simulink model "KP_Nikolaev_v27"  (R2021a)
settings: Solver=VariableStepAuto  StartTime=0.0  StopTime=50  RelTol=0.05
undefined symbols (not defined in the file): Angle, D11, Delta, Magnitude
libraries: spsThreePhaseBreakerLib x25, spsThreePhaseSeriesRLCLoadLib x15, spsSeriesRLCBranchLib x15, slrealtimeutilitieslib x14, slrealtimeiplib x13, spsThreePhaseVIMeasurementLib x6, spsCurrentMeasurementLib x3, spsPLLLib x3, spsVoltageMeasurementLib x3, spsExcitationSystemLib x2, spsSteamTurbineandGovernorLib x2, spsSynchronousMachinepuStandardLib x2
settings Model: Creator=kirill  LastModifiedBy=Артур
settings SolverCC: AlgebraicLoopSolver=TrustRegion
settings DebuggingCC: UnconnectedInputMsg=none  UnconnectedOutputMsg=none  UnconnectedLineMsg=none  SFMachineParentedDataDiag=warning

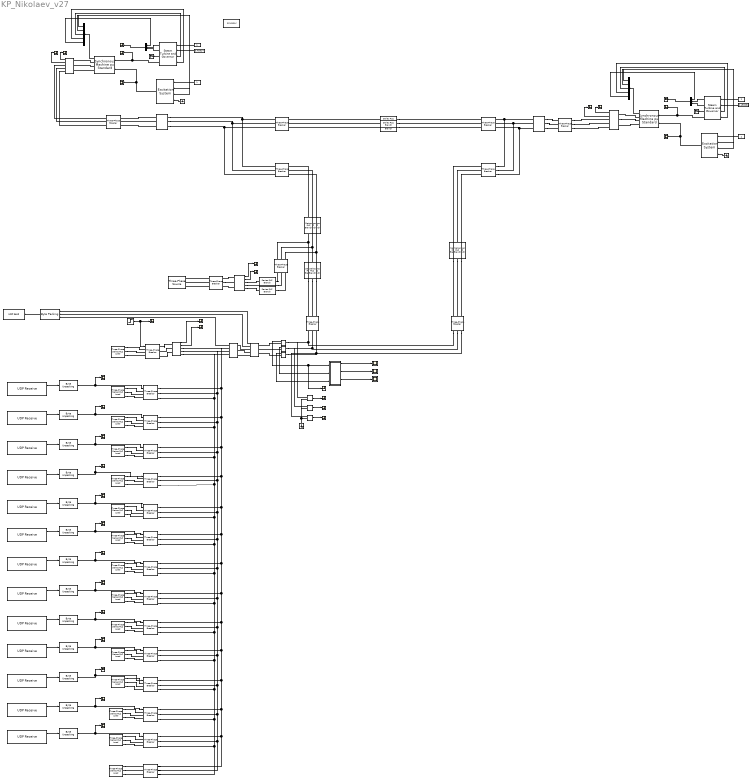
== system KP_Nikolaev_v27 ==
  A2 2 : spsCurrentMeasurementLib/Current Measurement  PhasorSimulation=off  OutputType=Magnitude-Angle  PSBequivalent=0
  A2 3 : spsCurrentMeasurementLib/Current Measurement  PhasorSimulation=off  OutputType=Magnitude-Angle  PSBequivalent=0
  A2 4 : spsCurrentMeasurementLib/Current Measurement  PhasorSimulation=off  OutputType=Magnitude-Angle  PSBequivalent=0
  Breaker0 : spsThreePhaseBreakerLib/Three-Phase Breaker  InitialState=open  SwitchA=on  SwitchB=on  SwitchC=on  SwitchTimes="[1/60  5/60]"  External=on  BreakerResistance=0.01  SnubberResistance=1e6  SnubberCapacitance=inf  Measurements=None
  Breaker{1..13} (13 alike) : spsThreePhaseBreakerLib/Three-Phase Breaker  InitialState=closed  SwitchA=on  SwitchB=on  SwitchC=on  SwitchTimes="[1/60  5/60]"  External=on  BreakerResistance=0.01  SnubberResistance=1e6  SnubberCapacitance=inf  Measurements=None
  Breaker{15..22,25..27} (11 alike) : spsThreePhaseBreakerLib/Three-Phase Breaker  InitialState=closed  SwitchA=off  SwitchB=off  SwitchC=off  SwitchTimes="[1/60  5/60]"  External=off  BreakerResistance=0.01  SnubberResistance=1e6  SnubberCapacitance=inf  Measurements=None
  Bus Creator1 : BusCreator  Inputs=3
  Bus Creator2 : BusCreator  Inputs=3
  Bus Selector1 : BusSelector  OutputSignals="dq0 components.Stator voltage  vd (pu),dq0 components.Stator voltage  vq (pu),Mechanical.Rotor speed  wm  (pu),Mechanical.Rotor angle deviation  d_theta (rad),Mechanical.Rotor speed deviation  dw (pu)"
  Bus Selector2 : BusSelector  OutputSignals="dq0 components.Stator voltage  vd (pu),dq0 components.Stator voltage  vq (pu),Mechanical.Rotor speed  wm  (pu),Mechanical.Rotor angle deviation  d_theta (rad),Mechanical.Rotor speed deviation  dw (pu)"
  Byte Packing : slrealtimeutilitieslib/Byte Packing  MaskPackedDataType=double  MaskUnpackedDataTypes={'double' 'double' 'double'}  MaskAlignment=1
  Byte Unpacking{,1..11,13} (13 alike) : slrealtimeutilitieslib/Byte Unpacking  MaskUnpackedDataTypes={'double'}  MaskUnpackedDataSizes={[1]}  MaskAlignment=1
      settings: SourceProductBaseCode=XP
  Constant{1..2,4..5} (4 alike) : Constant
  Constant3 : Constant  Value=0.458031
  Constant6 : Constant  Value=0.45914
  Excitation System1 : spsExcitationSystemLib/Excitation System  tr=10e-3  reg=[ 19, 0.001 ]  exc=[ 3, 0 ]  tgr=[ 0, 0 ]  damp=[ 0.001, 0.1 ]  sat=[ 0, 0 ]  lim=[ -11.5, 11.5, 0 ]  v0=[1,2.39309]
      settings: SourceProductBaseCode=PS
  Excitation System2 : spsExcitationSystemLib/Excitation System  tr=10e-3  reg=[ 19, 0.001 ]  exc=[ 3, 0 ]  tgr=[ 0, 0 ]  damp=[ 0.001, 0.1 ]  sat=[ 0, 0 ]  lim=[ -11.5, 11.5, 0 ]  v0=[1,2.39644]
      settings: SourceProductBaseCode=PS
  FreqIa : Scope
  FreqIb : Scope
  FreqIc : Scope
  Ground1 : Ground
  Ground10 : spsGroundLib/Ground  LConnTagsString=a
  Ground2 : Ground
  P0 : spsThreePhaseSeriesRLCLoadLib/Three-Phase Series RLC Load  LConnTagsString=A|B|C  Configuration=Y (grounded)  NominalVoltage=230000  Vabc=[1e3 1e3 1e3]  Vabcp=[1e3 1e3 1e3]  NominalFrequency=50  UnbalancedPower=off  ActivePower=(52.264e+06)*1.5  InductivePower=(40.21e+06)*1.5  CapacitivePower=0  Pabc=[10e3 9e3 11e3]  QLabc=[100 90 110]  QCabc=[100 90 110]  Pabcp=[10e3 9e3 11e3]  QLabcp=[100 90 110]  QCabcp=[100 90 110]  Measurements=None  LoadType=constant PQ
  P{1..11} (11 alike) : spsThreePhaseSeriesRLCLoadLib/Three-Phase Series RLC Load  LConnTagsString=A|B|C  Configuration=Y (grounded)  NominalVoltage=(230000)*0.901184  Vabc=[1e3 1e3 1e3]  Vabcp=[1e3 1e3 1e3]  NominalFrequency=50  UnbalancedPower=off  ActivePower=4325000  InductivePower=3244000  CapacitivePower=0  Pabc=[10e3 9e3 11e3]  QLabc=[100 90 110]  QCabc=[100 90 110]  Pabcp=[10e3 9e3 11e3]  QLabcp=[100 90 110]  QCabcp=[100 90 110]  Measurements=None  LoadType=constant PQ
  P12 : spsThreePhaseSeriesRLCLoadLib/Three-Phase Series RLC Load  LConnTagsString=A|B|C  Configuration=Y (grounded)  NominalVoltage=(230000)*0.901182  Vabc=[1e3 1e3 1e3]  Vabcp=[1e3 1e3 1e3]  NominalFrequency=50  UnbalancedPower=off  ActivePower=9531000  InductivePower=7149000  CapacitivePower=0  Pabc=[10e3 9e3 11e3]  QLabc=[100 90 110]  QCabc=[100 90 110]  Pabcp=[10e3 9e3 11e3]  QLabcp=[100 90 110]  QCabcp=[100 90 110]  Measurements=None  LoadType=constant PQ
  P13 : spsThreePhaseSeriesRLCLoadLib/Three-Phase Series RLC Load  LConnTagsString=A|B|C  Configuration=Y (grounded)  NominalVoltage=(230000)*0.901182  Vabc=[1e3 1e3 1e3]  Vabcp=[1e3 1e3 1e3]  NominalFrequency=50  UnbalancedPower=off  ActivePower=9531000  InductivePower=7149000  CapacitivePower=0  Pabc=[10e3 9e3 11e3]  QLabc=[100 90 110]  QCabc=[100 90 110]  Pabcp=[10e3 9e3 11e3]  QLabcp=[100 90 110]  QCabcp=[100 90 110]  Measurements=None  LoadType=constant PQ
  P14 : spsThreePhaseSeriesRLCLoadLib/Three-Phase Series RLC Load  LConnTagsString=A|B|C  Configuration=Y (grounded)  NominalVoltage=(230000)*0.901163  Vabc=[1e3 1e3 1e3]  Vabcp=[1e3 1e3 1e3]  NominalFrequency=50  UnbalancedPower=off  ActivePower=52422500  InductivePower=39317000  CapacitivePower=0  Pabc=[10e3 9e3 11e3]  QLabc=[100 90 110]  QCabc=[100 90 110]  Pabcp=[10e3 9e3 11e3]  QLabcp=[100 90 110]  QCabcp=[100 90 110]  Measurements=None  LoadType=constant PQ
  Scope{1..17,19..20,22..30,32..35} (32 alike) : Scope
  Series RLC Branch{1..3,18..20} (6 alike) : spsSeriesRLCBranchLib/Series RLC Branch  LConnTagsString=__new0  RConnTagsString=__new0  BranchType=RLC  Resistance=12.45  Inductance=70.187e-3  SetiL0=off  InitialCurrent=0  Capacitance=4.07436e-3  Setx0=off  InitialVoltage=0  Measurements=None
  Series RLC Branch{4..6,9..11} (6 alike) : spsSeriesRLCBranchLib/Series RLC Branch  LConnTagsString=__new0  RConnTagsString=__new0  BranchType=RLC  Resistance=6.225  Inductance=35.0935e-3  SetiL0=off  InitialCurrent=0  Capacitance=2.03718e-3  Setx0=off  InitialVoltage=0  Measurements=None
  Series RLC Branch21 : spsSeriesRLCBranchLib/Series RLC Branch  LConnTagsString=__new0  RConnTagsString=__new0  BranchType=RLC  Resistance=9.75  Inductance=70e-3  SetiL0=off  InitialCurrent=0  Capacitance=4e-3  Setx0=off  InitialVoltage=0  Measurements=None
  Series RLC Branch7 : spsSeriesRLCBranchLib/Series RLC Branch  LConnTagsString=__new0  RConnTagsString=__new0  BranchType=RLC  Resistance=9.75  Inductance=70e-3  SetiL0=off  InitialCurrent=0  Capacitance=4.07436e-3  Setx0=off  InitialVoltage=0  Measurements=None
  Series RLC Branch8 : spsSeriesRLCBranchLib/Series RLC Branch  LConnTagsString=__new0  RConnTagsString=__new0  BranchType=RLC  Resistance=9.75  Inductance=70e-3  SetiL0=off  InitialCurrent=0  Capacitance=4e-3  Setx0=off  InitialVoltage=0  Measurements=None
  Steam Turbine and Governor1 : spsSteamTurbineandGovernorLib/Steam Turbine and Governor  gentype=Tandem-compound (single mass)  reg1="[ 5 0.05  0 ]"  reg2="[ 0.001  0.15 ]"  reg3="[ -0.1 0.1  0  10.496]"  N=3000  turb1="[ 0  40 20  2 ]"  turb2="[ 0.5   0.5   0.0  0 ]"  HA="[  1.5498   0.24894  0  0 ]"  KA="[  83.47  42.702  0  0 ]"  DA="[  0.3104  0.05  0  0 ]*8"  ini1=0.502501  ini2=[0.429327,-63.9543]
      settings: SourceProductBaseCode=PS
  Steam Turbine and Governor2 : spsSteamTurbineandGovernorLib/Steam Turbine and Governor  gentype=Tandem-compound (single mass)  reg1="[ 5 0.05  0 ]"  reg2="[ 0.001  0.15 ]"  reg3="[ -0.1 0.1  0  10.496]"  N=3000  turb1="[ 0  40 20  2 ]"  turb2="[ 0.5   0.5   0.0  0 ]"  HA="[  1.5498   0.24894  0  0 ]"  KA="[  83.47  42.702  0  0 ]"  DA="[  0.3104  0.05  0  0 ]*8"  ini1=0.503721  ini2=[0.429327,-63.9543]
      settings: SourceProductBaseCode=PS
  Step : Step  Time=10  SampleTime=0  VectorParams1D=off
  Subsystem : Subsystem
  Synchronous Machine1 : spsSynchronousMachinepuStandardLib/Synchronous Machine pu Standard  PresetModel=No  MechanicalLoad=Mechanical power Pm  ShowDetailedParameters=on  RotorType=Round  Units=per unit standard parameters  MeasurementBus=off  NominalParameters=[78.75e+06 10.5e+03 50]  Reactances1=[ 1.915, 0.275, 0.203, 0.82, 0.65, 0.25, 0.15 ]  Reactances2=[1.71 0.172 0.119 0.59 0.23 0.1]  dAxisTimeConstants=Short-circuit  qAxisTimeConstants=Short-circuit  TimeConstants1="[ 4.4849  0.0681  0.1  ]"  TimeConstants2=[ 8.0, 0.03, 1.0, 0.07 ]  TimeConstants3="[  4.49  0.0681  0.0513  ]"  TimeConstants4=[ 8.0, 0.03, 0.3371, 0.0295 ]  TimeConstants5=[ 1.01, 0.053, 0.1 ]  TimeConstants6=[ 1.3201, 0.023, 1.0, 0.07 ]  TimeConstants7=[1.42 0.0908 0.132]  TimeConstants8=[ 1.85, 0.126, 0.212, 0.169 ]  StatorResistance=0.037875  Mechanical=[0.1028 0.02056 1]  PolePairs=20  InitialConditions=[0 -77.2339 0.794531 0.794531 0.794531 -54.7923 -174.792 65.2077 2.39309]  SetSaturation=on  Saturation=[0.6404,0.7127,0.8441,0.9214,0.9956,1.082,1.19,1.316,1.457;0.7,0.7698,0.8872,0.9466,0.9969,1.046,1.1,1.151,1.201]  LoadFlowParameters=[2 63000000 0 0 0]  TsPowergui=0  TsBlock=-1  IterativeModel=Trapezoidal non iterative  IterativeDiscreteModel=Trapezoidal robust  BusType=swing  Pref=63000000  Qref=47250000  Qmin=-Inf  Qmax=Inf  PLF=0  QLF=0
      settings: SourceProductBaseCode=PS
  Synchronous Machine2 : spsSynchronousMachinepuStandardLib/Synchronous Machine pu Standard  PresetModel=No  MechanicalLoad=Mechanical power Pm  ShowDetailedParameters=on  RotorType=Round  Units=per unit standard parameters  MeasurementBus=off  NominalParameters=[78.75e+06 10.5e+03 50]  Reactances1=[ 1.915, 0.275, 0.203, 0.82, 0.65, 0.25, 0.15 ]  Reactances2=[1.71 0.172 0.119 0.59 0.23 0.1]  dAxisTimeConstants=Short-circuit  qAxisTimeConstants=Short-circuit  TimeConstants1="[ 4.4849  0.0681  0.1  ]"  TimeConstants2=[ 8.0, 0.03, 1.0, 0.07 ]  TimeConstants3="[  4.49  0.0681  0.0513  ]"  TimeConstants4=[ 8.0, 0.03, 0.3371, 0.0295 ]  TimeConstants5=[ 1.01, 0.053, 0.1 ]  TimeConstants6=[ 1.3201, 0.023, 1.0, 0.07 ]  TimeConstants7=[1.42 0.0908 0.132]  TimeConstants8=[ 1.85, 0.126, 0.212, 0.169 ]  StatorResistance=0.037875  Mechanical=[0.1028 0.02056 1]  PolePairs=20  InitialConditions=[0 -77.2182 0.796369 0.796369 0.796369 -54.7923 -174.792 65.2077 2.39644]  SetSaturation=on  Saturation=[0.6404,0.7127,0.8441,0.9214,0.9956,1.082,1.19,1.316,1.457;0.7,0.7698,0.8872,0.9466,0.9969,1.046,1.1,1.151,1.201]  LoadFlowParameters=[2 63000000 0 0 0]  TsPowergui=0  TsBlock=-1  IterativeModel=Trapezoidal non iterative  IterativeDiscreteModel=Trapezoidal robust  BusType=swing  Pref=63000000  Qref=47250000  Qmin=-Inf  Qmax=Inf  PLF=0  QLF=0
      settings: SourceProductBaseCode=PS
  Terminator1 : Terminator
  Terminator2 : Terminator
  Three-Phase Measurement 1 : spsThreePhaseVIMeasurementLib/Three-Phase V-I Measurement  VoltageMeasurement=phase-to-phase  SetLabelV=off  LabelV=Vabc  Vpu=off  VpuLL=off  CurrentMeasurement=no  SetLabelI=off  LabelI=Iabc  Ipu=off  Pbase=100e6  Vbase=115e3  OutputType=Complex  PhasorSimulation=off  PSBequivalent=0
  Three-Phase Measurement 2 : spsThreePhaseVIMeasurementLib/Three-Phase V-I Measurement  VoltageMeasurement=phase-to-phase  SetLabelV=off  LabelV=Vabc  Vpu=off  VpuLL=off  CurrentMeasurement=yes  SetLabelI=off  LabelI=Iabc  Ipu=off  Pbase=100e6  Vbase=500e3  OutputType=Complex  PhasorSimulation=off  PSBequivalent=0
  Three-Phase Measurement 4 : spsThreePhaseVIMeasurementLib/Three-Phase V-I Measurement  VoltageMeasurement=phase-to-ground  SetLabelV=off  LabelV=Vabc  Vpu=off  VpuLL=off  CurrentMeasurement=yes  SetLabelI=off  LabelI=Iabc  Ipu=off  Pbase=100e6  Vbase=115e3  OutputType=Complex  PhasorSimulation=off  PSBequivalent=0
  Three-Phase Transformer (Two Windings)1 : spsThreePhaseTransformerTwoWindingsLib/Three-Phase Transformer (Two Windings)  Winding1Connection=Y  Winding2Connection=Delta (D11)  CoreType=Three single-phase transformers  SetSaturation=off  Hysteresis=off  DataFile='hysteresis'  SetInitialFlux=off  Measurements=None  UNITS=SI  NominalPower=[ 80e6 , 50 ]  Winding1=[10500 0.00882 0.001123]  Winding2=[2.3e+05 11.616 1.479]  Rm=2205  Lm=7.0187  L0=0.5  Saturation=[0 0;4.6657 32.747;1944 41.48]  InitialFluxes=[ 0.8 , -0.8 , 0.7 ]  BreakLoop=on  DiscreteSolver=Trapezoidal iterative  DataType=on  TransfoNumber=1
  Three-Phase Transformer (Two Windings)2 : spsThreePhaseTransformerTwoWindingsLib/Three-Phase Transformer (Two Windings)  Winding1Connection=Y  Winding2Connection=Delta (D11)  CoreType=Three single-phase transformers  SetSaturation=off  Hysteresis=off  DataFile='hysteresis'  SetInitialFlux=off  Measurements=None  UNITS=SI  NominalPower=[ 80e6 , 50 ]  Winding1=[10500 0.00882 0.001123]  Winding2=[2.3e+05 11.616 1.479]  Rm=2205  Lm=7.0187  L0=0.5  Saturation=[0 0;4.6657 32.747;1944 41.48]  InitialFluxes=[ 0.8 , -0.8 , 0.7 ]  BreakLoop=on  DiscreteSolver=Trapezoidal iterative  DataType=on  TransfoNumber=1
  Three-Phase V-I Measurement1 : spsThreePhaseVIMeasurementLib/Three-Phase V-I Measurement  VoltageMeasurement=phase-to-phase  SetLabelV=off  LabelV=Vabc  Vpu=off  VpuLL=off  CurrentMeasurement=yes  SetLabelI=off  LabelI=Iabc  Ipu=off  Pbase=100e6  Vbase=10.5e3  OutputType=Complex  PhasorSimulation=off  PSBequivalent=0
  Three-Phase V-I Measurement2 : spsThreePhaseVIMeasurementLib/Three-Phase V-I Measurement  VoltageMeasurement=phase-to-phase  SetLabelV=off  LabelV=Vabc  Vpu=off  VpuLL=off  CurrentMeasurement=yes  SetLabelI=off  LabelI=Iabc  Ipu=off  Pbase=100e6  Vbase=10.5e3  OutputType=Complex  PhasorSimulation=off  PSBequivalent=0
  Three-Phase V-I Measurement4 : spsThreePhaseVIMeasurementLib/Three-Phase V-I Measurement  VoltageMeasurement=phase-to-ground  SetLabelV=off  LabelV=Vabc  Vpu=off  VpuLL=off  CurrentMeasurement=yes  SetLabelI=off  LabelI=Iabc  Ipu=off  Pbase=100e6  Vbase=500e3  OutputType=Complex  PhasorSimulation=off  PSBequivalent=0
  Three-Phase Source1 : spsThreePhaseSourceLib/Three-Phase Source  InternalConnection=Yg  VoltagePhases=off  Voltage=230000  PhaseAngle=0  Voltage_phases=[25e3 25e3 25e3]/sqrt(3)  PhaseAngles_phases=[0 -120 +120]  Frequency=50  NonIdealSource=on  SpecifyImpedance=off  Resistance=5  Inductance=1e-03  ShortCircuitLevel=100e6  BaseVoltage=230000  XRratio=7  BusType=swing  Pref=0  Qref=0  Prefabc=[10e3, 10e3, 10e3]  Qrefabc=[0, 0, 0]  Qmin=0  Qmax=0
  UDP Receive1 : slrealtimeiplib/UDP Receive  useHostTargetConn=on  ipAddress='localhost'  localPort=9002  rcvWidth=8  rcvFmAny=on  fmAddress=10.10.10.10  sampleTime=10e-5
      settings: SourceProductBaseCode=XP
  UDP Receive10 : slrealtimeiplib/UDP Receive  useHostTargetConn=on  ipAddress='localhost'  localPort=9011  rcvWidth=8  rcvFmAny=on  fmAddress=10.10.10.10  sampleTime=10e-5
      settings: SourceProductBaseCode=XP
  UDP Receive11 : slrealtimeiplib/UDP Receive  useHostTargetConn=on  ipAddress='localhost'  localPort=9012  rcvWidth=8  rcvFmAny=on  fmAddress=10.10.10.10  sampleTime=10e-5
      settings: SourceProductBaseCode=XP
  UDP Receive12 : slrealtimeiplib/UDP Receive  useHostTargetConn=on  ipAddress='localhost'  localPort=9013  rcvWidth=8  rcvFmAny=on  fmAddress=10.10.10.10  sampleTime=10e-5
      settings: SourceProductBaseCode=XP
  UDP Receive14 : slrealtimeiplib/UDP Receive  useHostTargetConn=on  ipAddress='localhost'  localPort=9001  rcvWidth=8  rcvFmAny=on  fmAddress=10.10.10.10  sampleTime=10e-5
      settings: SourceProductBaseCode=XP
  UDP Receive2 : slrealtimeiplib/UDP Receive  useHostTargetConn=on  ipAddress='localhost'  localPort=9003  rcvWidth=8  rcvFmAny=on  fmAddress=10.10.10.10  sampleTime=10e-5
      settings: SourceProductBaseCode=XP
  UDP Receive3 : slrealtimeiplib/UDP Receive  useHostTargetConn=on  ipAddress='localhost'  localPort=9004  rcvWidth=8  rcvFmAny=on  fmAddress=10.10.10.10  sampleTime=10e-5
      settings: SourceProductBaseCode=XP
  UDP Receive4 : slrealtimeiplib/UDP Receive  useHostTargetConn=on  ipAddress='localhost'  localPort=9005  rcvWidth=8  rcvFmAny=on  fmAddress=10.10.10.10  sampleTime=10e-5
      settings: SourceProductBaseCode=XP
  UDP Receive5 : slrealtimeiplib/UDP Receive  useHostTargetConn=on  ipAddress='localhost'  localPort=9006  rcvWidth=8  rcvFmAny=on  fmAddress=10.10.10.10  sampleTime=10e-5
      settings: SourceProductBaseCode=XP
  UDP Receive6 : slrealtimeiplib/UDP Receive  useHostTargetConn=on  ipAddress='localhost'  localPort=9007  rcvWidth=8  rcvFmAny=on  fmAddress=10.10.10.10  sampleTime=10e-5
      settings: SourceProductBaseCode=XP
  UDP Receive7 : slrealtimeiplib/UDP Receive  useHostTargetConn=on  ipAddress='localhost'  localPort=9008  rcvWidth=8  rcvFmAny=on  fmAddress=10.10.10.10  sampleTime=10e-5
      settings: SourceProductBaseCode=XP
  UDP Receive8 : slrealtimeiplib/UDP Receive  useHostTargetConn=on  ipAddress='localhost'  localPort=9009  rcvWidth=8  rcvFmAny=on  fmAddress=10.10.10.10  sampleTime=10e-5
      settings: SourceProductBaseCode=XP
  UDP Receive9 : slrealtimeiplib/UDP Receive  useHostTargetConn=on  ipAddress='localhost'  localPort=9010  rcvWidth=8  rcvFmAny=on  fmAddress=10.10.10.10  sampleTime=10e-5
      settings: SourceProductBaseCode=XP
  UDP Send : dspnetwork/UDP Send  remoteURL='localhost'  remotePort=9090  localURL='0.0.0.0'  localPortSource=Automatically determine  localPort=-1  sendBufferSize=24  sampletime=-1  blockPlatform=[]  separateLengthPort=0
  V11 : spsVoltageMeasurementLib/Voltage Measurement  PhasorSimulation=off  OutputType=Complex  PSBequivalent=0
  V22 : spsVoltageMeasurementLib/Voltage Measurement  PhasorSimulation=off  OutputType=Complex  PSBequivalent=0
  V33 : spsVoltageMeasurementLib/Voltage Measurement  PhasorSimulation=off  OutputType=Complex  PSBequivalent=0
  powergui : spspowerguiLib/powergui  Priority=1  SimulationMode=Discrete  SampleTime=0.00025  frequency=60  Iterations=1000  frequencyindice=50  Pbase=100e6  ErrMax=1e-4  UnitsV=V  UnitsW=W  buscounter=0  FunctionMessages=off  echomessages=off  EnableUseOfTLC=off  CurrentSourceSwitches=off  DisableSnubberDevices=off  DisableRonSwitches=off  DisableVfSwitches=off  DisplayEquations=off  AutomaticDiscreteSolvers=off  SolverType=Tustin/Backward Euler (TBE)  Interpol=off  ExternalGateDelay=off  methode=off  Ts=100  x0status=blocks  SPID=on  SwTol=0  HookPort=off  NonlinearTolerance=1e-4  nMaxIteration=100  ContinueOnMaxIteration=off  RestoreLinks=warning  ResistiveCurrentMeasurement=off  Frange=[0:2:500]  Ylog=off  Xlog=on  ShowGrid=off  save=off  variable=ZData  structure=0  ZoomFFT=off  StartTime=0.0  cycles=1  DisplayStyle=1  fundamental=60  FreqAxis=off  MaxFrequency=1000  frequencyindicesteady=1  RmsSteady=1  display=off
  wires:
  A2 2/1 -> Scope35/1, Subsystem/1(In1)
  A2 3/1 -> Subsystem/2(In2)
  A2 4/1 -> Subsystem/3(In3)
  Subsystem/1(Freq) -> FreqIa/1
  Subsystem/3(Freq1) -> FreqIb/1
  Subsystem/5(Freq2) -> FreqIc/1
  Bus Selector2/3 -> Steam Turbine and Governor2/3  "<Rotor speed  wm  (pu)>"
  Bus Selector2/4 -> Steam Turbine and Governor2/4  "<Rotor angle deviation  d_theta (rad)>"
  Bus Creator1/1 -> Scope3/1
  Steam Turbine and Governor2/2 -> Bus Creator1/3
  Constant5/1 -> Steam Turbine and Governor2/1
  Three-Phase V-I Measurement1/2 -> Scope4/1
  Bus Selector2/5 -> Bus Creator1/1  "<Rotor speed deviation  dw (pu)>"
  Constant4/1 -> Excitation System2/1
  Ground2/1 -> Excitation System2/4
  Bus Selector2/2 -> Excitation System2/3  "<Stator voltage  vq (pu)>"
  Steam Turbine and Governor2/4 -> Synchronous Machine2/1, Scope6/1
  Excitation System2/1 -> Synchronous Machine2/2, Scope1/1
  Bus Selector2/1 -> Excitation System2/2  "<Stator voltage  vd (pu)>"
  Steam Turbine and Governor2/1 -> Bus Creator1/2
  Three-Phase V-I Measurement1/1 -> Scope2/1
  Synchronous Machine2/1 -> Bus Selector2/1
  Constant6/1 -> Steam Turbine and Governor2/2
  Steam Turbine and Governor2/3 -> Terminator2/1
  Steam Turbine and Governor1/3 -> Terminator1/1
  Excitation System1/1 -> Synchronous Machine1/2, Scope10/1
  Bus Selector1/3 -> Steam Turbine and Governor1/3  "<Rotor speed  wm  (pu)>"
  Three-Phase V-I Measurement2/2 -> Scope8/1
  Constant2/1 -> Steam Turbine and Governor1/1
  Synchronous Machine1/1 -> Bus Selector1/1
  Three-Phase V-I Measurement2/1 -> Scope5/1
  Bus Creator2/1 -> Scope7/1
  Bus Selector1/5 -> Bus Creator2/1  "<Rotor speed deviation  dw (pu)>"
  Bus Selector1/2 -> Excitation System1/3  "<Stator voltage  vq (pu)>"
  Constant1/1 -> Excitation System1/1
  Steam Turbine and Governor1/1 -> Bus Creator2/2
  Steam Turbine and Governor1/2 -> Bus Creator2/3
  Steam Turbine and Governor1/4 -> Synchronous Machine1/1, Scope9/1
  Ground1/1 -> Excitation System1/4
  Bus Selector1/4 -> Steam Turbine and Governor1/4  "<Rotor angle deviation  d_theta (rad)>"
  Bus Selector1/1 -> Excitation System1/2  "<Stator voltage  vd (pu)>"
  Constant3/1 -> Steam Turbine and Governor1/2
  Step/1 -> Breaker0/1, Scope13/1
  Three-Phase Measurement 2/1 -> Scope20/1
  Three-Phase Measurement 2/2 -> Scope16/1
  Three-Phase V-I Measurement4/2 -> Scope11/1
  Three-Phase V-I Measurement4/1 -> Scope12/1
  Three-Phase Measurement 4/1 -> Byte Packing/1
  Three-Phase Measurement 1/1 -> Byte Packing/3
  Byte Packing/1 -> UDP Send/1
  Three-Phase Measurement 4/2 -> Byte Packing/2
  Byte Unpacking5/1 -> Breaker7/1, Scope26/1
  Byte Unpacking13/1 -> Breaker1/1, Scope17/1
  Byte Unpacking10/1 -> Breaker12/1, Scope14/1
  UDP Receive10/1 -> Byte Unpacking9/1
  Byte Unpacking11/1 -> Breaker13/1, Scope15/1
  Byte Unpacking6/1 -> Breaker8/1, Scope27/1
  UDP Receive2/1 -> Byte Unpacking1/1
  UDP Receive1/1 -> Byte Unpacking/1
  Byte Unpacking/1 -> Breaker2/1, Scope19/1
  UDP Receive4/1 -> Byte Unpacking3/1
  UDP Receive6/1 -> Byte Unpacking5/1
  UDP Receive9/1 -> Byte Unpacking8/1
  UDP Receive14/1 -> Byte Unpacking13/1
  Byte Unpacking9/1 -> Breaker11/1, Scope30/1
  UDP Receive12/1 -> Byte Unpacking11/1
  UDP Receive7/1 -> Byte Unpacking6/1
  UDP Receive5/1 -> Byte Unpacking4/1
  Byte Unpacking3/1 -> Breaker5/1, Scope24/1
  UDP Receive3/1 -> Byte Unpacking2/1
  Byte Unpacking8/1 -> Breaker10/1, Scope29/1
  Byte Unpacking1/1 -> Breaker3/1, Scope22/1
  UDP Receive11/1 -> Byte Unpacking10/1
  Byte Unpacking7/1 -> Breaker9/1, Scope28/1
  Byte Unpacking4/1 -> Breaker6/1, Scope25/1
  Byte Unpacking2/1 -> Breaker4/1, Scope23/1
  UDP Receive8/1 -> Byte Unpacking7/1
  V11/1 -> Scope32/1
  V22/1 -> Scope33/1
  V33/1 -> Scope34/1
  connections:
  Breaker1/RConn3 -- Three-Phase Measurement 2/RConn3 -- Three-Phase Measurement 1/RConn3 -- Breaker2/RConn3 -- Breaker3/RConn3 -- Breaker4/RConn3 -- Breaker5/RConn3 -- Breaker6/RConn3 -- Breaker7/RConn3 -- Breaker8/RConn3 -- Breaker9/RConn3 -- Breaker10/RConn3 -- Breaker11/RConn3 -- Breaker12/RConn3 -- Breaker15/RConn3 -- Breaker13/RConn3
  Breaker1/RConn2 -- Three-Phase Measurement 1/RConn2 -- Three-Phase Measurement 2/RConn2 -- Breaker2/RConn2 -- Breaker3/RConn2 -- Breaker4/RConn2 -- Breaker5/RConn2 -- Breaker6/RConn2 -- Breaker7/RConn2 -- Breaker8/RConn2 -- Breaker9/RConn2 -- Breaker10/RConn2 -- Breaker11/RConn2 -- Breaker12/RConn2 -- Breaker15/RConn2 -- Breaker13/RConn2
  Breaker15/RConn1 -- Three-Phase Measurement 2/RConn1 -- Three-Phase Measurement 1/RConn1 -- Breaker1/RConn1 -- Breaker2/RConn1 -- Breaker3/RConn1 -- Breaker4/RConn1 -- Breaker5/RConn1 -- Breaker6/RConn1 -- Breaker7/RConn1 -- Breaker8/RConn1 -- Breaker9/RConn1 -- Breaker10/RConn1 -- Breaker11/RConn1 -- Breaker12/RConn1 -- Breaker13/RConn1
  P2/LConn3 -- Breaker2/LConn3
  P2/LConn2 -- Breaker2/LConn2
  P2/LConn1 -- Breaker2/LConn1
  P3/LConn2 -- Breaker3/LConn2
  P3/LConn3 -- Breaker3/LConn3
  P3/LConn1 -- Breaker3/LConn1
  P4/LConn3 -- Breaker4/LConn3
  P4/LConn1 -- Breaker4/LConn1
  P5/LConn2 -- Breaker5/LConn2
  P4/LConn2 -- Breaker4/LConn2
  P5/LConn3 -- Breaker5/LConn3
  P5/LConn1 -- Breaker5/LConn1
  P9/LConn3 -- Breaker9/LConn3
  P6/LConn1 -- Breaker6/LConn1
  P7/LConn2 -- Breaker7/LConn2
  P8/LConn1 -- Breaker8/LConn1
  P9/LConn2 -- Breaker9/LConn2
  P7/LConn3 -- Breaker7/LConn3
  P9/LConn1 -- Breaker9/LConn1
  P6/LConn2 -- Breaker6/LConn2
  P6/LConn3 -- Breaker6/LConn3
  P7/LConn1 -- Breaker7/LConn1
  P8/LConn3 -- Breaker8/LConn3
  P8/LConn2 -- Breaker8/LConn2
  P10/LConn1 -- Breaker10/LConn1
  P11/LConn2 -- Breaker11/LConn2
  P11/LConn3 -- Breaker11/LConn3
  P10/LConn2 -- Breaker10/LConn2
  P10/LConn3 -- Breaker10/LConn3
  P11/LConn1 -- Breaker11/LConn1
  P12/LConn1 -- Breaker12/LConn1
  P12/LConn2 -- Breaker12/LConn2
  P12/LConn3 -- Breaker12/LConn3
  P13/LConn3 -- Breaker13/LConn3
  P13/LConn2 -- Breaker13/LConn2
  P13/LConn1 -- Breaker13/LConn1
  P14/LConn1 -- Breaker15/LConn1
  P14/LConn3 -- Breaker15/LConn3
  P14/LConn2 -- Breaker15/LConn2
  P1/LConn1 -- Breaker1/LConn1
  P1/LConn2 -- Breaker1/LConn2
  P1/LConn3 -- Breaker1/LConn3
  Breaker17/LConn1 -- Three-Phase Transformer (Two Windings)2/RConn1 -- Breaker16/LConn1
  Breaker17/LConn2 -- Three-Phase Transformer (Two Windings)2/RConn2 -- Breaker16/LConn2
  Breaker17/LConn3 -- Three-Phase Transformer (Two Windings)2/RConn3 -- Breaker16/LConn3
  Breaker18/RConn3 -- Three-Phase Transformer (Two Windings)1/RConn3 -- Breaker19/RConn3
  Breaker18/RConn2 -- Three-Phase Transformer (Two Windings)1/RConn2 -- Breaker19/RConn2
  Breaker18/RConn1 -- Three-Phase Transformer (Two Windings)1/RConn1 -- Breaker19/RConn1
  Breaker21/RConn3 -- A2 4/LConn1 -- V33/LConn1 -- Breaker20/LConn3
  Breaker21/RConn1 -- A2 2/LConn1 -- V11/LConn1 -- Breaker20/LConn1
  Breaker21/RConn2 -- A2 3/LConn1 -- V22/LConn1 -- Breaker20/LConn2
  Three-Phase Transformer (Two Windings)1/LConn1 -- Breaker26/LConn1
  Three-Phase Transformer (Two Windings)1/LConn2 -- Breaker26/LConn2
  Three-Phase Transformer (Two Windings)1/LConn3 -- Breaker26/LConn3
  Series RLC Branch18/RConn1 -- Breaker19/LConn1
  Series RLC Branch18/LConn1 -- Breaker16/RConn1
  Series RLC Branch20/LConn1 -- Breaker16/RConn2
  Series RLC Branch19/LConn1 -- Breaker16/RConn3
  Series RLC Branch20/RConn1 -- Breaker19/LConn2
  Series RLC Branch19/RConn1 -- Breaker19/LConn3
  Series RLC Branch3/LConn1 -- Breaker21/LConn2
  Series RLC Branch2/LConn1 -- Breaker21/LConn3
  Series RLC Branch1/LConn1 -- Breaker21/LConn1
  Series RLC Branch1/RConn1 -- Breaker18/LConn1
  Series RLC Branch3/RConn1 -- Breaker18/LConn2
  Series RLC Branch2/RConn1 -- Breaker18/LConn3
  Series RLC Branch11/RConn1 -- Breaker27/LConn1 -- Series RLC Branch5/LConn1
  Series RLC Branch9/RConn1 -- Breaker27/LConn2 -- Series RLC Branch4/LConn1
  Series RLC Branch6/RConn1 -- Breaker27/LConn3 -- Series RLC Branch10/LConn1
  Series RLC Branch10/RConn1 -- Breaker17/RConn3
  Series RLC Branch5/RConn1 -- Breaker17/RConn1
  Series RLC Branch4/RConn1 -- Breaker17/RConn2
  Series RLC Branch6/LConn1 -- Breaker20/RConn3
  Series RLC Branch9/LConn1 -- Breaker20/RConn2
  Series RLC Branch11/LConn1 -- Breaker20/RConn1
  A2 2/RConn1 -- Three-Phase Measurement 4/LConn1
  A2 3/RConn1 -- Three-Phase Measurement 4/LConn2
  A2 4/RConn1 -- Three-Phase Measurement 4/LConn3
  V33/LConn2 -- V11/LConn2 -- V22/LConn2 -- Ground10/LConn1
  Three-Phase Measurement 4/RConn1 -- Three-Phase Measurement 1/LConn1
  Three-Phase Measurement 4/RConn2 -- Three-Phase Measurement 1/LConn2
  Three-Phase Measurement 4/RConn3 -- Three-Phase Measurement 1/LConn3
  Synchronous Machine2/RConn1 -- Three-Phase V-I Measurement1/LConn1
  Three-Phase Transformer (Two Windings)2/LConn2 -- Breaker25/RConn2
  Breaker25/LConn1 -- Three-Phase V-I Measurement1/RConn1
  Breaker25/LConn3 -- Three-Phase V-I Measurement1/RConn3
  Three-Phase Transformer (Two Windings)2/LConn3 -- Breaker25/RConn3
  Three-Phase Transformer (Two Windings)2/LConn1 -- Breaker25/RConn1
  Breaker25/LConn2 -- Three-Phase V-I Measurement1/RConn2
  Synchronous Machine2/RConn2 -- Three-Phase V-I Measurement1/LConn2
  Synchronous Machine2/RConn3 -- Three-Phase V-I Measurement1/LConn3
  Breaker26/RConn1 -- Three-Phase V-I Measurement2/RConn1
  Three-Phase V-I Measurement2/LConn2 -- Synchronous Machine1/RConn2
  Breaker26/RConn2 -- Three-Phase V-I Measurement2/RConn2
  Breaker26/RConn3 -- Three-Phase V-I Measurement2/RConn3
  Synchronous Machine1/RConn3 -- Three-Phase V-I Measurement2/LConn3
  Synchronous Machine1/RConn1 -- Three-Phase V-I Measurement2/LConn1
  Three-Phase Measurement 2/LConn3 -- Breaker0/RConn3
  P0/LConn1 -- Breaker0/LConn1
  P0/LConn2 -- Breaker0/LConn2
  Three-Phase Measurement 2/LConn1 -- Breaker0/RConn1
  P0/LConn3 -- Breaker0/LConn3
  Three-Phase Measurement 2/LConn2 -- Breaker0/RConn2
  Three-Phase V-I Measurement4/RConn3 -- Series RLC Branch8/LConn1
  Three-Phase V-I Measurement4/LConn3 -- Breaker22/RConn3
  Series RLC Branch8/RConn1 -- Breaker27/RConn3
  Series RLC Branch7/RConn1 -- Breaker27/RConn1
  Three-Phase V-I Measurement4/LConn1 -- Breaker22/RConn1
  Breaker22/LConn1 -- Three-Phase Source1/RConn1
  Breaker22/RConn2 -- Three-Phase V-I Measurement4/LConn2
  Three-Phase V-I Measurement4/RConn1 -- Series RLC Branch7/LConn1
  Breaker22/LConn3 -- Three-Phase Source1/RConn3
  Three-Phase V-I Measurement4/RConn2 -- Series RLC Branch21/LConn1
  Series RLC Branch21/RConn1 -- Breaker27/RConn2
  Breaker22/LConn2 -- Three-Phase Source1/RConn2

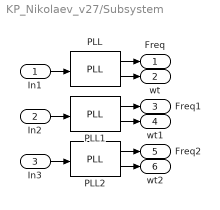
== system KP_Nikolaev_v27/Subsystem ==
  In1 : Inport
  In2 : Inport  Port=2
  In3 : Inport  Port=3
  PLL : spsPLLLib/PLL  Fmin=45  Par_Init=[0, 50]  ParK=[180, 3200, 1]  TcD=1e-4  MaxRateChangeFreq=12  FilterCutOffFreq=25  Ts=0  AGC=on
      settings: SourceProductBaseCode=PS
  PLL1 : spsPLLLib/PLL  Fmin=45  Par_Init=[0, 50]  ParK=[180, 3200, 1]  TcD=1e-4  MaxRateChangeFreq=12  FilterCutOffFreq=25  Ts=0  AGC=on
      settings: SourceProductBaseCode=PS
  PLL2 : spsPLLLib/PLL  Fmin=45  Par_Init=[0, 50]  ParK=[180, 3200, 1]  TcD=1e-4  MaxRateChangeFreq=12  FilterCutOffFreq=25  Ts=0  AGC=on
      settings: SourceProductBaseCode=PS
  Freq : Outport
  wt : Outport  Port=2
  Freq1 : Outport  Port=3
  wt1 : Outport  Port=4
  Freq2 : Outport  Port=5
  wt2 : Outport  Port=6
  wires:
  In2/1 -> PLL1/1
  In3/1 -> PLL2/1
  PLL/1 -> Freq/1
  PLL/2 -> wt/1
  PLL1/2 -> wt1/1
  PLL2/2 -> wt2/1
  PLL1/1 -> Freq1/1
  In1/1 -> PLL/1
  PLL2/1 -> Freq2/1
